simulink model "Segway_sim"  (R2016a)
settings: Solver=ode4  StartTime=0.0  StopTime=Tsim  FixedStep=1/fs  RelTol=1e-3
values from neighbouring files (symbols this model uses):
  c1 = Mp*l^2 + Ip    (= 20)    [Check_psi.m]    (also in Gradient_Check.m; Segway.m; Segway_tau.m)
  c10 = -Mp*l    (= -10)    [Check_psi.m]    (also in Gradient_Check.m; Segway.m; Segway_tau.m)
  c2 = -2*km*ke/(R*r)    (= -8.1)    [Check_psi.m]    (also in Gradient_Check.m; Segway.m = -0.1; Segway_tau.m)
  c3 = 2*km/R    (= 1.8)    [Check_psi.m]    (also in Gradient_Check.m; Segway.m = 20; Segway_tau.m)
  c4 = Mp*g*l    (= 98.1)    [Check_psi.m]    (also in Gradient_Check.m; Segway.m; Segway_tau.m)
  c5 = -Mp*l    (= -10)    [Check_psi.m]    (also in Gradient_Check.m; Segway.m; Segway_tau.m)
  c6 = 2*km/(R*r)    (= 9)    [Check_psi.m]    (also in Gradient_Check.m; Segway.m = 100; Segway_tau.m)
  c7 = 2*Mw + 2*Iw/r^2 + Mp    (= 16)    [Check_psi.m]    (also in Gradient_Check.m; Segway.m; Segway_tau.m)
  c8 = 2*km*ke/(R*r^2)    (= 40.5)    [Check_psi.m]    (also in Gradient_Check.m; Segway.m = 0.5; Segway_tau.m)
  c9 = Mp*l    (= 10)    [Check_psi.m]    (also in Gradient_Check.m; Segway.m; Segway_tau.m)
  x0 = [0;0;pi+10*pi/180;0;0]    [Check_psi.m]    (also in Gradient_Check.m = [0;0;10*pi/180;0;0]; Segway.m = [0;0;0;0]; Segway_tau.m = [-4;0;10*pi/180;0;0]; rk4.m = xnext)
settings Model: Creator=Marcin  LastModifiedBy=Marcin
settings GRTTargetCC: GeneratePreprocessorConditionals=Use local settings

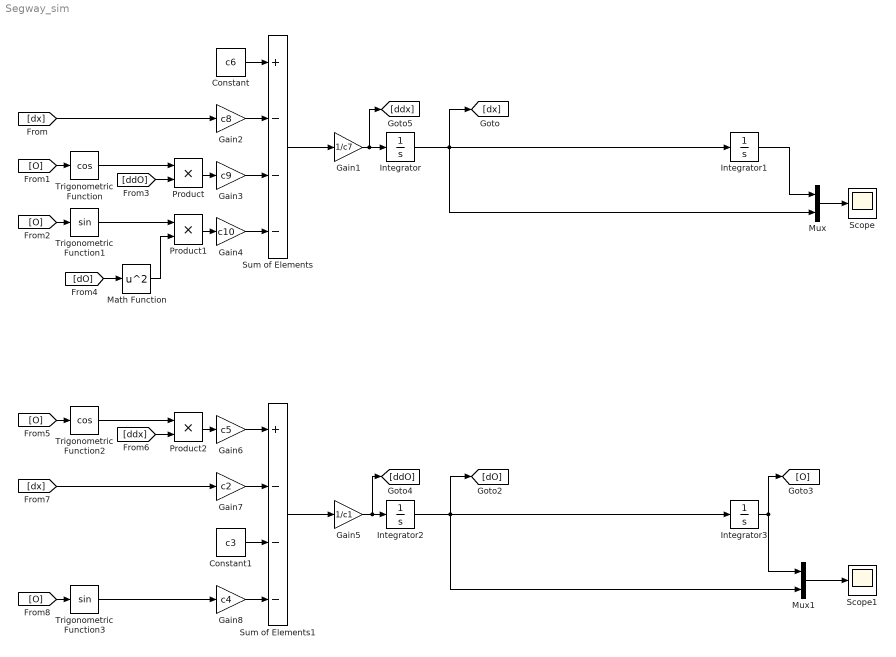
== system Segway_sim ==
  Constant : Constant  Value=c6
  Constant1 : Constant  Value=c3
  Gain1 : Gain  Gain=1/c7
  Gain2 : Gain  Gain=c8
  Gain3 : Gain  Gain=c9
  Gain4 : Gain  Gain=c10
  Gain5 : Gain  Gain=1/c1
  Gain6 : Gain  Gain=c5
  Gain7 : Gain  Gain=c2
  Gain8 : Gain  Gain=c4
  Integrator : Integrator  InitialCondition=x0(2)
  Integrator1 : Integrator  InitialCondition=x0(1)
  Integrator2 : Integrator  InitialCondition=x0(4)
  Integrator3 : Integrator  InitialCondition=x0(3)
  Math Function : Math  Operator=square  SaturateOnIntegerOverflow=on
  Mux : Mux  Inputs=2
  Mux1 : Mux  Inputs=2
  Product : Product
  Product1 : Product
  Product2 : Product
  Scope : Scope
  Scope1 : Scope
  Sum of Elements : Sum  Inputs=+---
  Sum of Elements1 : Sum  Inputs=+---
  Trigonometric Function : Trigonometry  Operator=cos
  Trigonometric Function1 : Trigonometry
  Trigonometric Function2 : Trigonometry  Operator=cos
  Trigonometric Function3 : Trigonometry
  wires:
  Integrator/1 -> Mux/2, [dx], Integrator1/1
  Integrator2/1 -> Mux1/2, [dO], Integrator3/1
  Gain1/1 -> [ddx], Integrator/1
  Gain5/1 -> [ddO], Integrator2/1
  Sum of Elements/1 -> Gain1/1
  Constant/1 -> Sum of Elements/1
  Gain2/1 -> Sum of Elements/2
  Integrator3/1 -> Mux1/1, [O]
  [dx] -> Gain2/1
  Gain3/1 -> Sum of Elements/3
  Gain4/1 -> Sum of Elements/4
  [O] -> Trigonometric Function/1
  [O] -> Trigonometric Function1/1
  Product/1 -> Gain3/1
  Trigonometric Function/1 -> Product/1
  Trigonometric Function1/1 -> Product1/1
  [ddO] -> Product/2
  Math Function/1 -> Product1/2
  [dO] -> Math Function/1
  Product1/1 -> Gain4/1
  Sum of Elements1/1 -> Gain5/1
  Gain6/1 -> Sum of Elements1/1
  [O] -> Trigonometric Function2/1
  Product2/1 -> Gain6/1
  Trigonometric Function2/1 -> Product2/1
  [ddx] -> Product2/2
  Gain7/1 -> Sum of Elements1/2
  [dx] -> Gain7/1
  Constant1/1 -> Sum of Elements1/3
  [O] -> Trigonometric Function3/1
  Trigonometric Function3/1 -> Gain8/1
  Gain8/1 -> Sum of Elements1/4
  Integrator1/1 -> Mux/1
  Mux/1 -> Scope/1
  Mux1/1 -> Scope1/1
